simulink model "etc_r2v_subs"  (R2022b)
settings: Solver=FixedStepDiscrete  StartTime=0.0  StopTime=10.0  RelTol=1e-3  EnableMultiTasking=on
PreLoadFcn:
  | % Input data
  | t = linspace(0,10,101)';
  | u = linspace(0,pi/2,101)';
  | 
  | % Conversion factor
  | degConv = 180/pi;
settings Model: Creator=jrivitus  LastModifiedBy=bensweet
settings SolverCC: AlgebraicLoopSolver=TrustRegion
settings DataIOCC: LimitDataPoints=on  LoadExternalInput=on  SaveFormat=Array  ReturnWorkspaceOutputs=off
settings OptimizationCC: ExpressionDepthLimit=2147483647  LifeSpan=inf
settings DebuggingCC: UnconnectedInputMsg=warning  UnconnectedOutputMsg=warning  UnconnectedLineMsg=warning  PregeneratedLibrarySubsystemCodeDiagnostic=none  SFMachineParentedDataDiag=warning
settings HardwareCC: ProdBitPerPointer=32  ProdBitPerSizeT=32  ProdBitPerPtrDiffT=32  ProdLargestAtomicFloat=None  ProdIntDivRoundTo=Undefined  ProdEndianess=Unspecified  ProdWordSize=32  ProdHWDeviceType=32-bit Generic
settings ModelReferenceCC: EnableRefExpFcnMdlSchedulingChecks=on  PropagateSignalLabelsOutOfModel=off
settings SFSimCC: SimUseLocalCustomCode=off
settings RTWCC: RTWUseLocalCustomCode=off  DLArmComputeVersion=19.05
settings CodeAppCC: StateflowObjectComments=on
settings GRTTargetCC: TargetLangStandard=C89/C90 (ANSI)  CombineOutputUpdateFcns=off  GRTInterface=on
settings ConfigComp: CovMetricSettings=dw  CovSaveCumulativeToWorkspaceVar=on  CovSaveSingleToWorkspaceVar=on  CovExternalEMLEnable=off  CovSFcnEnable=off

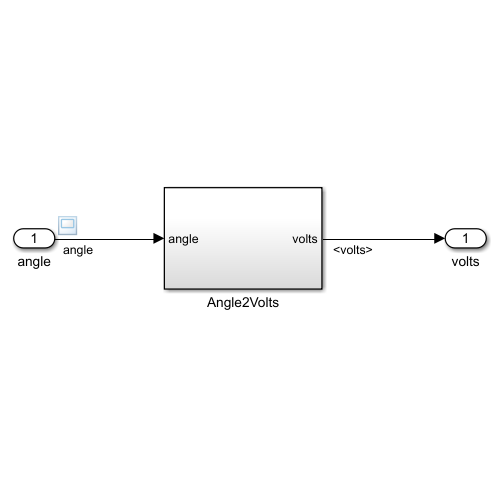
[thumbnail: Simulink's stored preview of the top-level diagram]
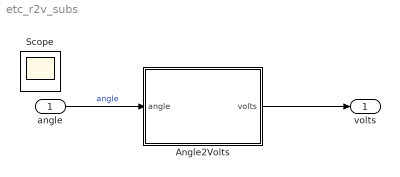
== system etc_r2v_subs ==
  angle : Inport
  Angle2Volts : Subsystem
  volts : Outport  VectorParamsAs1DForOutWhenUnconnected=off
  Scope : Scope
  wires:
  Angle2Volts/1(volts) -> volts/1
  angle/1 -> Angle2Volts/1(angle)  "angle"

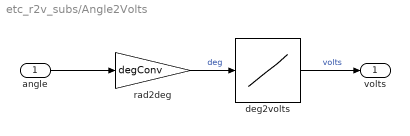
== system etc_r2v_subs/Angle2Volts ==
  angle : Inport
  deg2volts : Lookup_n-D  NumberOfTableDimensions=1  BreakpointsForDimension1=[0 90]  Table=[0.5 4.5]  RndMeth=Simplest
  rad2deg : Gain  Gain=degConv  SaturateOnIntegerOverflow=on  OutDataTypeStr=Inherit: Same as input  ParamDataTypeStr=Inherit: Same as input
  volts : Outport  VectorParamsAs1DForOutWhenUnconnected=off
  wires:
  angle/1 -> rad2deg/1
  deg2volts/1 -> volts/1  "volts"
  rad2deg/1 -> deg2volts/1  "deg"
